simulink model "Testerr"  (R2024a)
settings: Solver=FixedStepAuto  StartTime=0.0  StopTime=inf  RelTol=1e-3  EnableMultiTasking=on
undefined symbols (not defined in the file): DiscIntNeverNeededParam
libraries: stm32f4xxblockslib x15, mcbpositiondecoderlib x4, stm32blockslib x3, simulink x1, mcbcontrolslib x1
settings Model: SimulationMode=external  Creator=wsl  LastModifiedBy=wsl
settings SolverCC: AllowMultiTaskInputOutput=on  AutoInsertRateTranBlk=on  InsertRTBMode=Never (minimum delay)
settings OptimizationCC: EnhancedBackFolding=on  PassReuseOutputArgsAs=Individual arguments  ZeroExternalMemoryAtStartup=off  ZeroInternalMemoryAtStartup=off  MaxStackSize=64  OptimizeBlockOrder=speed  DifferentSizesBufferReuse=on  OptimizationCustomize=off  EfficientTunableParamExpr=on
settings DebuggingCC: MultiTaskDSMMsg=none  TasksWithSamePriorityMsg=none  ParameterPrecisionLossMsg=none  ParameterTunabilityLossMsg=error
settings HardwareCC: ProdBitPerPointer=32  ProdBitPerSizeT=32  ProdBitPerPtrDiffT=32  ProdLargestAtomicInteger=Long  ProdLargestAtomicFloat=Double  ProdWordSize=32  ProdLongLongMode=on  ProdHWDeviceType=ARM Compatible->ARM Cortex-M
settings SFSimCC: MATLABDynamicMemAlloc=off
settings RTWCC: Description=Embedded Coder  SystemTargetFile=ert.tlc  HardwareBoard=STM32F4xx Based  TemplateMakefile=ert_default_tmf  Toolchain=GNU Tools for ARM Embedded Processors
settings CodeAppCC: ForceParamTrailComments=on  IgnoreCustomStorageClasses=off  OperatorAnnotations=on  SimulinkDataObjDesc=on  SFDataObjDesc=on  InsertBlockDesc=on
settings ERTTargetCC: TargetLangStandard=C99 (ISO)  CodeReplacementLibrary=ARM Cortex-M  ExtModeTransport=3  ExtModeStaticAlloc=on  ExtModeStaticAllocSize=2048  ExtModeMexFile=ext_xcp  ExtModeIntrfLevel=Level2 - Open

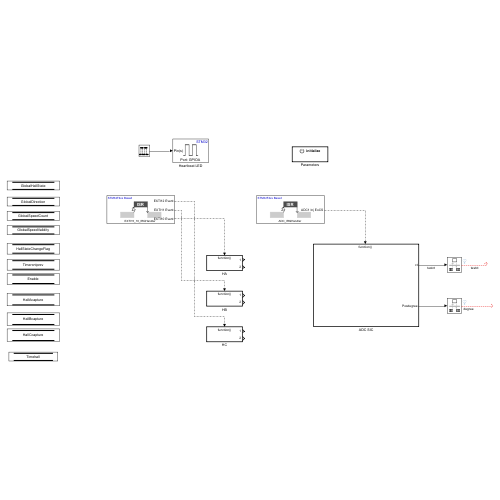
[thumbnail: Simulink's stored preview of the top-level diagram]
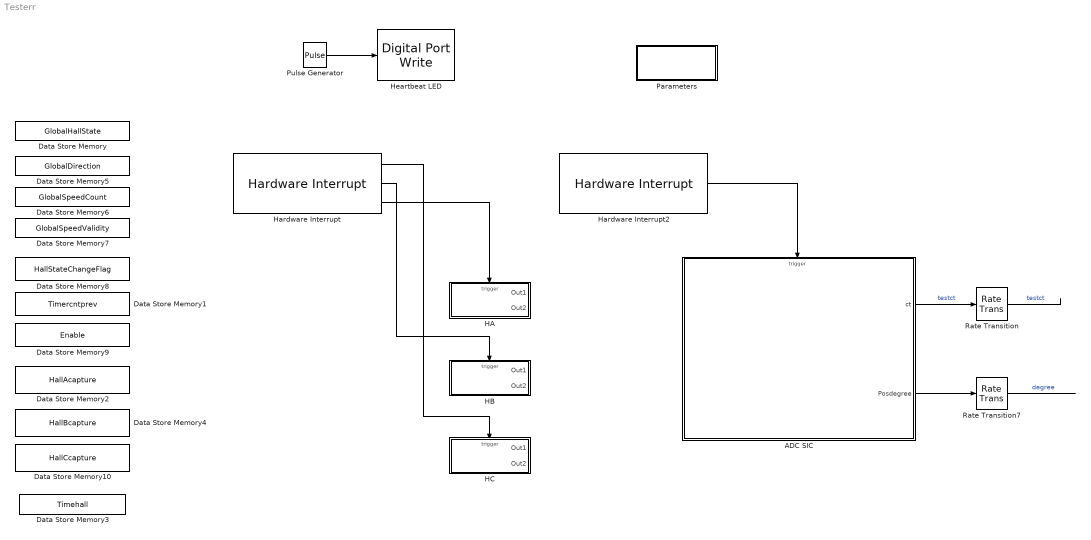
== system Testerr ==
  ADC SIC : Subsystem  TreatAsAtomicUnit=on
  Data Store Memory : DataStoreMemory  DataStoreName=GlobalHallState  WriteAfterWriteMsg=warning  ShowAdditionalParam=off
  Data Store Memory1 : DataStoreMemory  DataStoreName=Timercntprev  WriteAfterWriteMsg=warning  ShowAdditionalParam=off
  Data Store Memory10 : DataStoreMemory  DataStoreName=HallCcapture  WriteAfterWriteMsg=warning  ShowAdditionalParam=off
  Data Store Memory2 : DataStoreMemory  DataStoreName=HallAcapture  WriteAfterWriteMsg=warning  ShowAdditionalParam=off
  Data Store Memory3 : DataStoreMemory  DataStoreName=Timehall  WriteAfterWriteMsg=warning  ShowAdditionalParam=off
  Data Store Memory4 : DataStoreMemory  DataStoreName=HallBcapture  WriteAfterWriteMsg=warning  ShowAdditionalParam=off
  Data Store Memory5 : DataStoreMemory  DataStoreName=GlobalDirection  WriteAfterWriteMsg=warning  ShowAdditionalParam=off
  Data Store Memory6 : DataStoreMemory  DataStoreName=GlobalSpeedCount  WriteAfterWriteMsg=warning  ShowAdditionalParam=off
  Data Store Memory7 : DataStoreMemory  DataStoreName=GlobalSpeedValidity  WriteAfterWriteMsg=warning  ShowAdditionalParam=off
  Data Store Memory8 : DataStoreMemory  DataStoreName=HallStateChangeFlag  WriteAfterWriteMsg=warning  ShowAdditionalParam=off
  Data Store Memory9 : DataStoreMemory  DataStoreName=Enable  WriteAfterWriteMsg=warning  ShowAdditionalParam=off
  HA : Subsystem  TreatAsAtomicUnit=on
  HB : Subsystem  TreatAsAtomicUnit=on
  HC : Subsystem  TreatAsAtomicUnit=on
  Hardware Interrupt : stm32f4xxblockslib/Hardware Interrupt  ISRGroup=External interrupts (EXTI)  ISRName=EXTI15_10_IRQHandler  ISRNumber=55  EventsList={ 'off', 'EXTI15 Event', '1'; 'off', 'EXTI14 Event', '2'; 'off', 'EXTI13 Event', '3'; 'on', 'EXTI12 Event', '4'; 'on', 'EXTI11 Event', '5'; 'on', 'EXTI10 Event', '6'; 'off', 'Custom event', '7' }  SelectedEvents={'EXTI12 Event','EXTI11 Event','EXTI10 Event'}  TaskPriority=30  DisablePreemption=on  ClearInterruptFlagsAtEndOfEvent=off  InterruptDefinitionFile=$(TARGET_ROOT)/registry/interrupts/STM32F4xxBased_interrupts.xml  HardwareBoard=STM32F4xx Based  EnableSimPort=off
  Hardware Interrupt2 : stm32f4xxblockslib/Hardware Interrupt  ISRGroup=Analog to digital converter (ADC)  ISRName=ADC_IRQHandler  ISRNumber=33  EventsList={ 'off', 'ADC1 OVR', '1'; 'off', 'ADC1 Reg EoCS', '2'; 'on', 'ADC1 Inj EoCS', '3'; 'off', 'ADC1 Watchdog', '4'; 'off', 'ADC2 OVR', '5'; 'off', 'ADC2 Reg EoCS', '6'; 'off', 'ADC2 Inj EoCS', '7'; 'off', 'ADC2 Watchdog', '8'; 'off', 'ADC3 OVR', '9'; 'off', 'ADC3 Reg EoCS', '10'; 'off', 'ADC3 Inj EoCS', '11'; 'off', 'ADC3 Watchdog', '12'; 'off', 'Custom event', '13' }  SelectedEvents={'ADC1 Inj EoCS'}  TaskPriority=30  DisablePreemption=on  ClearInterruptFlagsAtEndOfEvent=off  InterruptDefinitionFile=$(TARGET_ROOT)/registry/interrupts/STM32F4xxBased_interrupts.xml  HardwareBoard=STM32F4xx Based  EnableSimPort=off
  Heartbeat LED : stm32f4xxblockslib/Digital Port Write  PortName=GPIOA  PinNumber=[5]  ReadOperation=off  IOAsArray=on  EnableSimPort=off
  Parameters : Subsystem  TreatAsAtomicUnit=on
  Pulse Generator : DiscretePulseGenerator  Period=10  PulseWidth=5  SampleTime=0.1
  Rate Transition : RateTransition  Deterministic=off  OutPortSampleTime=1e-3
  Rate Transition7 : RateTransition  Deterministic=off  OutPortSampleTime=1e-3
  wires:
  Pulse Generator/1 -> Heartbeat LED/1
  Hardware Interrupt/2 -> HB/Trigger
  Hardware Interrupt/3 -> HA/Trigger
  Hardware Interrupt/1 -> HC/Trigger
  Hardware Interrupt2/1 -> ADC SIC/Trigger
  ADC SIC/1(ct) -> Rate Transition/1  "testct"
  Rate Transition/1 -> ?  "testct"
  Rate Transition7/1 -> ?  "degree"
  ADC SIC/2(Posdegree) -> Rate Transition7/1

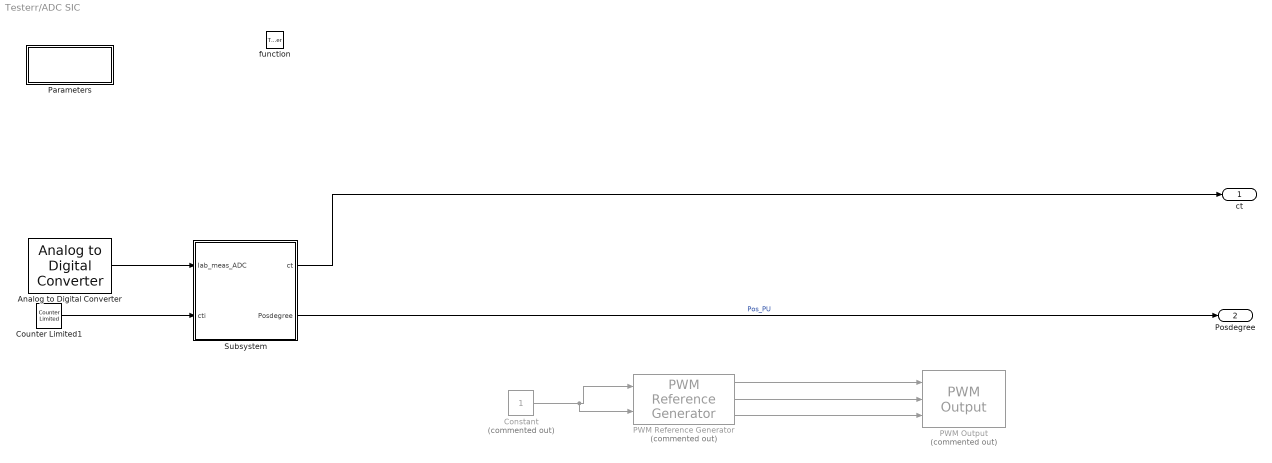
== system Testerr/ADC SIC ==
  function : TriggerPort  TriggerType=function-call  VariantControl=(inherit)
  Analog to Digital Converter : stm32f4xxblockslib/Analog to Digital Converter  ADCModule=ADC1  ConversionGroup=Injected  TriggerMode=Read results only  NumberOfConversions=3  EnableBufferConv=off  BufferLength=1  OutputStatus=off  SampleTime=-1  EnableSimPort=off
  Constant : Constant  Commented=on
  Counter Limited1 : simulink/Sources/Counter Limited  uplimit=20000  tsamp=-1
  PWM Output : stm32f4xxblockslib/PWM Output  Commented=on  TimerModule=TIM1  DutycycleUnits=Percentage  EnableChannel1=on  EnableChannel2=on  EnableChannel3=on  EnableChannel4=off  EnableCounterInput=off  EnableMainOutputInput=off  EnableFrequencyInput=off  SetRCAfterCE=on  OutputDirection=off  OutputMainOutputEnableStatus=off  SampleTime=0.1  EnableSimPort=off  EnableUpdateEvent=off  EnableCaptureCompare1Event=off  EnableCaptureCompare2Event=off  EnableCaptureCompare3Event=off  EnableCaptureCompare4Event=off  EnableTriggerEvent=off  EnableBreakEvent=off  ProcessorFamily=STM32F4  hoistedMaskSrc=ECSoC/ECSimCodegen/PWM Output
  PWM Reference Generator : mcbcontrolslib/PWM Reference Generator  Commented=on  inSignal=Valphabeta  modType=SVM: space vector modulation
      settings: LibrarySourceBlock=mcblib/Controls/Math Transforms/PWM Reference Generator
  Parameters : Subsystem  TreatAsAtomicUnit=on
  Subsystem : Subsystem
  ct : Outport
  Posdegree : Outport  Port=2
  wires:
  Analog to Digital Converter/1 -> Subsystem/1(Iab_meas_ADC)
  Counter Limited1/1 -> Subsystem/2(cti)
  Subsystem/1(ct) -> ct/1
  Subsystem/2(Posdegree) -> Posdegree/1  "Pos_PU"
  PWM Reference Generator/2 -> PWM Output/2
  PWM Reference Generator/1 -> PWM Output/1
  PWM Reference Generator/3 -> PWM Output/3
  Constant/1 -> PWM Reference Generator/2, PWM Reference Generator/1

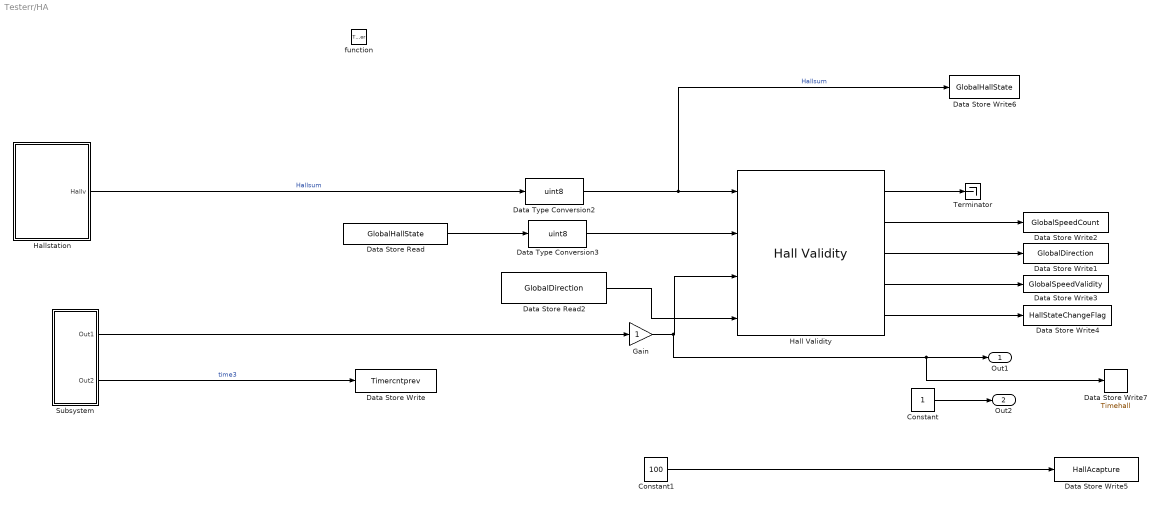
== system Testerr/HA ==
  function : TriggerPort  TriggerType=function-call  VariantControl=(inherit)
  Constant : Constant
  Constant1 : Constant  Value=100
  Data Store Read : DataStoreRead  DataStoreName=GlobalHallState  IndexOptions=Index vector (dialog)  Indices=1  OutputSizes=1
  Data Store Read2 : DataStoreRead  DataStoreName=GlobalDirection  IndexOptions=Index vector (dialog)  Indices=1  OutputSizes=1
  Data Store Write : DataStoreWrite  DataStoreName=Timercntprev  IndexOptions=Index vector (dialog)  Indices=1  OutputSizes=1
  Data Store Write1 : DataStoreWrite  DataStoreName=GlobalDirection  IndexOptions=Index vector (dialog)  Indices=1  OutputSizes=1
  Data Store Write2 : DataStoreWrite  DataStoreName=GlobalSpeedCount  IndexOptions=Index vector (dialog)  Indices=1  OutputSizes=1
  Data Store Write3 : DataStoreWrite  DataStoreName=GlobalSpeedValidity  IndexOptions=Index vector (dialog)  Indices=1  OutputSizes=1
  Data Store Write4 : DataStoreWrite  DataStoreName=HallStateChangeFlag  IndexOptions=Index vector (dialog)  Indices=1  OutputSizes=1
  Data Store Write5 : DataStoreWrite  DataStoreName=HallAcapture  IndexOptions=Index vector (dialog)  Indices=1  OutputSizes=1
  Data Store Write6 : DataStoreWrite  DataStoreName=GlobalHallState  IndexOptions=Index vector (dialog)  Indices=1  OutputSizes=1
  Data Store Write7 : DataStoreWrite  DataStoreName=Timehall  IndexOptions=Index vector (dialog)  Indices=1  OutputSizes=1
  Data Type Conversion2 : DataTypeConversion  OutDataTypeStr=uint8  SaturateOnIntegerOverflow=off  RndMeth=Floor
  Data Type Conversion3 : DataTypeConversion  OutDataTypeStr=uint8  SaturateOnIntegerOverflow=off  RndMeth=Floor
  Gain : Gain
  Hall Validity : mcbpositiondecoderlib/Hall Validity  hallSequence=ABC  sequence=[5,4,6,2,3,1]  CounterSize=32 bits
  Hallstation : Subsystem
  Subsystem : Subsystem
  Terminator : Terminator
  Out1 : Outport
  Out2 : Outport  Port=2
  wires:
  Hall Validity/2 -> Data Store Write2/1
  Hall Validity/3 -> Data Store Write1/1
  Data Store Read2/1 -> Hall Validity/4
  Hall Validity/1 -> Terminator/1
  Hall Validity/4 -> Data Store Write3/1
  Hall Validity/5 -> Data Store Write4/1
  Constant/1 -> Out2/1
  Data Store Read/1 -> Data Type Conversion3/1
  Hallstation/1(Hallv) -> Data Type Conversion2/1  "Hallsum"
  Data Type Conversion3/1 -> Hall Validity/2
  Subsystem/1(Out1) -> Gain/1
  Data Type Conversion2/1 -> Data Store Write6/1, Hall Validity/1  "Hallsum"
  Gain/1 -> Data Store Write7/1, Out1/1, Hall Validity/3
  Constant1/1 -> Data Store Write5/1
  Subsystem/2(Out2) -> Data Store Write/1  "time3"

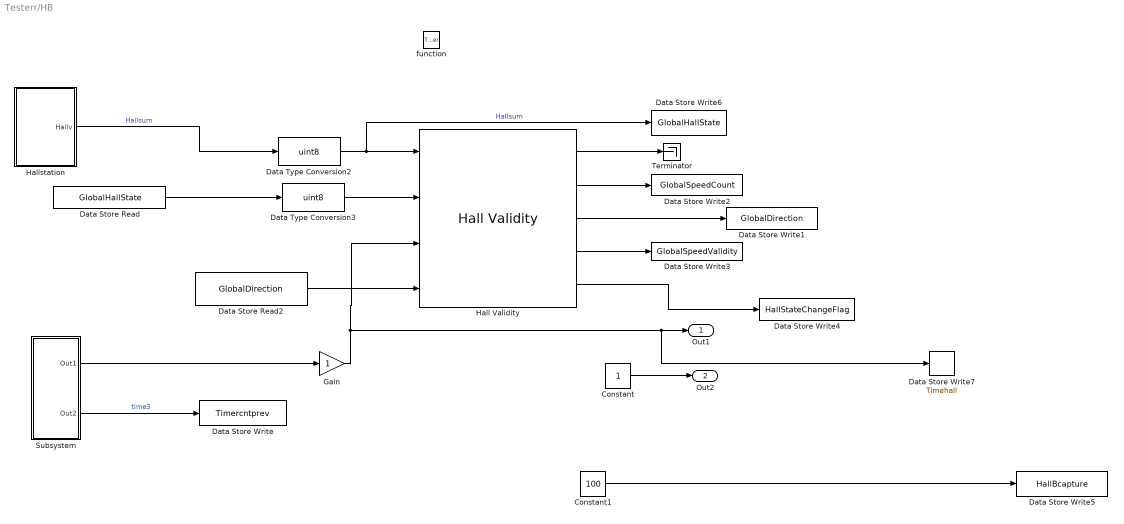
== system Testerr/HB ==
  function : TriggerPort  TriggerType=function-call  VariantControl=(inherit)
  Constant : Constant
  Constant1 : Constant  Value=100
  Data Store Read : DataStoreRead  DataStoreName=GlobalHallState  IndexOptions=Index vector (dialog)  Indices=1  OutputSizes=1
  Data Store Read2 : DataStoreRead  DataStoreName=GlobalDirection  IndexOptions=Index vector (dialog)  Indices=1  OutputSizes=1
  Data Store Write : DataStoreWrite  DataStoreName=Timercntprev  IndexOptions=Index vector (dialog)  Indices=1  OutputSizes=1
  Data Store Write1 : DataStoreWrite  DataStoreName=GlobalDirection  IndexOptions=Index vector (dialog)  Indices=1  OutputSizes=1
  Data Store Write2 : DataStoreWrite  DataStoreName=GlobalSpeedCount  IndexOptions=Index vector (dialog)  Indices=1  OutputSizes=1
  Data Store Write3 : DataStoreWrite  DataStoreName=GlobalSpeedValidity  IndexOptions=Index vector (dialog)  Indices=1  OutputSizes=1
  Data Store Write4 : DataStoreWrite  DataStoreName=HallStateChangeFlag  IndexOptions=Index vector (dialog)  Indices=1  OutputSizes=1
  Data Store Write5 : DataStoreWrite  DataStoreName=HallBcapture  IndexOptions=Index vector (dialog)  Indices=1  OutputSizes=1
  Data Store Write6 : DataStoreWrite  DataStoreName=GlobalHallState  IndexOptions=Index vector (dialog)  Indices=1  OutputSizes=1
  Data Store Write7 : DataStoreWrite  DataStoreName=Timehall  IndexOptions=Index vector (dialog)  Indices=1  OutputSizes=1
  Data Type Conversion2 : DataTypeConversion  OutDataTypeStr=uint8  SaturateOnIntegerOverflow=off  RndMeth=Floor
  Data Type Conversion3 : DataTypeConversion  OutDataTypeStr=uint8  SaturateOnIntegerOverflow=off  RndMeth=Floor
  Gain : Gain
  Hall Validity : mcbpositiondecoderlib/Hall Validity  hallSequence=ABC  sequence=[5,4,6,2,3,1]  CounterSize=32 bits
  Hallstation : Subsystem
  Subsystem : Subsystem
  Terminator : Terminator
  Out1 : Outport
  Out2 : Outport  Port=2
  wires:
  Hall Validity/2 -> Data Store Write2/1
  Hall Validity/3 -> Data Store Write1/1
  Data Store Read2/1 -> Hall Validity/4
  Hall Validity/1 -> Terminator/1
  Hall Validity/4 -> Data Store Write3/1
  Hall Validity/5 -> Data Store Write4/1
  Constant/1 -> Out2/1
  Hallstation/1(Hallv) -> Data Type Conversion2/1  "Hallsum"
  Data Type Conversion3/1 -> Hall Validity/2
  Subsystem/1(Out1) -> Gain/1
  Data Type Conversion2/1 -> Data Store Write6/1, Hall Validity/1  "Hallsum"
  Data Store Read/1 -> Data Type Conversion3/1
  Gain/1 -> Hall Validity/3, Data Store Write7/1, Out1/1
  Constant1/1 -> Data Store Write5/1
  Subsystem/2(Out2) -> Data Store Write/1  "time3"

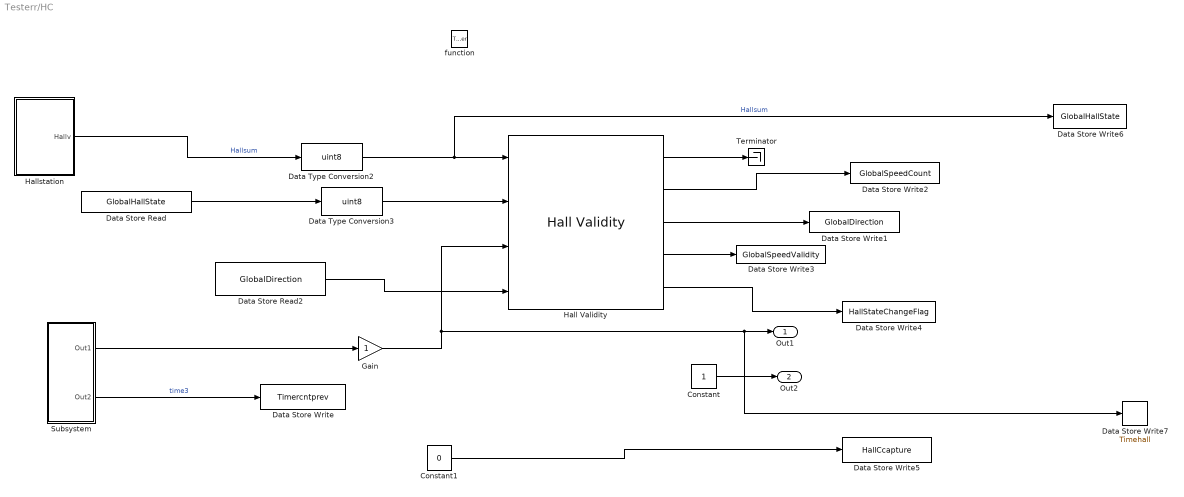
== system Testerr/HC ==
  function : TriggerPort  TriggerType=function-call  VariantControl=(inherit)
  Constant : Constant
  Constant1 : Constant  Value=0
  Data Store Read : DataStoreRead  DataStoreName=GlobalHallState  IndexOptions=Index vector (dialog)  Indices=1  OutputSizes=1
  Data Store Read2 : DataStoreRead  DataStoreName=GlobalDirection  IndexOptions=Index vector (dialog)  Indices=1  OutputSizes=1
  Data Store Write : DataStoreWrite  DataStoreName=Timercntprev  IndexOptions=Index vector (dialog)  Indices=1  OutputSizes=1
  Data Store Write1 : DataStoreWrite  DataStoreName=GlobalDirection  IndexOptions=Index vector (dialog)  Indices=1  OutputSizes=1
  Data Store Write2 : DataStoreWrite  DataStoreName=GlobalSpeedCount  IndexOptions=Index vector (dialog)  Indices=1  OutputSizes=1
  Data Store Write3 : DataStoreWrite  DataStoreName=GlobalSpeedValidity  IndexOptions=Index vector (dialog)  Indices=1  OutputSizes=1
  Data Store Write4 : DataStoreWrite  DataStoreName=HallStateChangeFlag  IndexOptions=Index vector (dialog)  Indices=1  OutputSizes=1
  Data Store Write5 : DataStoreWrite  DataStoreName=HallCcapture  IndexOptions=Index vector (dialog)  Indices=1  OutputSizes=1
  Data Store Write6 : DataStoreWrite  DataStoreName=GlobalHallState  IndexOptions=Index vector (dialog)  Indices=1  OutputSizes=1
  Data Store Write7 : DataStoreWrite  DataStoreName=Timehall  IndexOptions=Index vector (dialog)  Indices=1  OutputSizes=1
  Data Type Conversion2 : DataTypeConversion  OutDataTypeStr=uint8  SaturateOnIntegerOverflow=off  RndMeth=Floor
  Data Type Conversion3 : DataTypeConversion  OutDataTypeStr=uint8  SaturateOnIntegerOverflow=off  RndMeth=Floor
  Gain : Gain
  Hall Validity : mcbpositiondecoderlib/Hall Validity  hallSequence=ABC  sequence=[5,4,6,2,3,1]  CounterSize=32 bits
  Hallstation : Subsystem
  Subsystem : Subsystem
  Terminator : Terminator
  Out1 : Outport
  Out2 : Outport  Port=2
  wires:
  Hall Validity/2 -> Data Store Write2/1
  Hall Validity/3 -> Data Store Write1/1
  Data Store Read2/1 -> Hall Validity/4
  Hall Validity/1 -> Terminator/1
  Hall Validity/4 -> Data Store Write3/1
  Hall Validity/5 -> Data Store Write4/1
  Constant/1 -> Out2/1
  Hallstation/1(Hallv) -> Data Type Conversion2/1  "Hallsum"
  Data Store Read/1 -> Data Type Conversion3/1
  Subsystem/1(Out1) -> Gain/1
  Data Type Conversion3/1 -> Hall Validity/2
  Data Type Conversion2/1 -> Data Store Write6/1, Hall Validity/1  "Hallsum"
  Gain/1 -> Hall Validity/3, Data Store Write7/1, Out1/1
  Constant1/1 -> Data Store Write5/1
  Subsystem/2(Out2) -> Data Store Write/1  "time3"

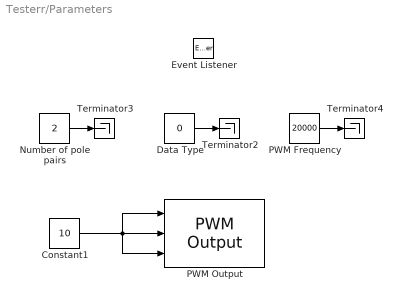
== system Testerr/Parameters ==
  Constant1 : Constant  Value=10  VectorParams1D=off
  Data Type : Constant  Value=0
  Event Listener : EventListener  DisableCoverage=on  EventName=reset
  Number of pole pairs : Constant  Value=2
  PWM Frequency : Constant  Value=20000
  PWM Output : stm32f4xxblockslib/PWM Output  TimerModule=TIM1  DutycycleUnits=Percentage  EnableChannel1=on  EnableChannel2=on  EnableChannel3=on  EnableChannel4=off  EnableCounterInput=off  EnableMainOutputInput=off  EnableFrequencyInput=off  SetRCAfterCE=on  OutputDirection=off  OutputMainOutputEnableStatus=off  SampleTime=0.1  EnableSimPort=off  EnableUpdateEvent=off  EnableCaptureCompare1Event=off  EnableCaptureCompare2Event=off  EnableCaptureCompare3Event=off  EnableCaptureCompare4Event=off  EnableTriggerEvent=off  EnableBreakEvent=off  ProcessorFamily=STM32F4  hoistedMaskSrc=ECSoC/ECSimCodegen/PWM Output
  Terminator2 : Terminator
  Terminator3 : Terminator
  Terminator4 : Terminator
  wires:
  PWM Frequency/1 -> Terminator4/1
  Number of pole pairs/1 -> Terminator3/1
  Data Type/1 -> Terminator2/1
  Constant1/1 -> PWM Output/3, PWM Output/2, PWM Output/1

== system Testerr/ADC SIC/Parameters ==
  Data Type : Constant  Value=0
  Event Listener : EventListener  DisableCoverage=on  EventName=reset
  Number of pole pairs : Constant  Value=4
  PWM Frequency : Constant  Value=20000
  Terminator2 : Terminator
  Terminator3 : Terminator
  Terminator4 : Terminator
  wires:
  PWM Frequency/1 -> Terminator4/1
  Number of pole pairs/1 -> Terminator3/1
  Data Type/1 -> Terminator2/1

== system Testerr/ADC SIC/Subsystem ==
  Iab_meas_ADC : Inport  OutDataTypeStr=uint16
  cti : Inport  Port=2
  Subsystem1 : Subsystem
  Terminator : Terminator
  ct : Outport
  Posdegree : Outport  Port=2
  wires:
  Iab_meas_ADC/1 -> Terminator/1
  Subsystem1/2(Posdegree) -> Posdegree/1
  Subsystem1/1(ct) -> ct/1
  cti/1 -> Subsystem1/1(cti)

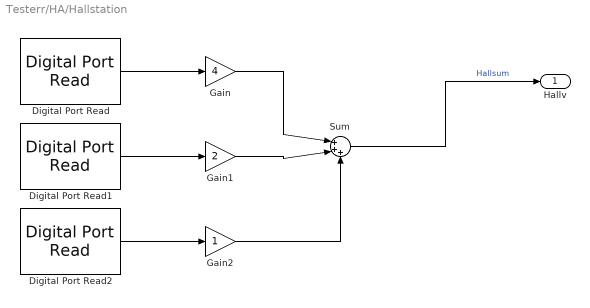
== system Testerr/HA/Hallstation ==
  Digital Port Read : stm32f4xxblockslib/Digital Port Read  PortName=GPIOC  PinNumber=[10]  ReadOperation=on  IOAsArray=on  SampleTime=-1  EnableSimPort=off
  Digital Port Read1 : stm32f4xxblockslib/Digital Port Read  PortName=GPIOC  PinNumber=[11]  ReadOperation=on  IOAsArray=on  SampleTime=-1  EnableSimPort=off
  Digital Port Read2 : stm32f4xxblockslib/Digital Port Read  PortName=GPIOC  PinNumber=[12]  ReadOperation=on  IOAsArray=on  SampleTime=-1  EnableSimPort=off
  Gain : Gain  Gain=4  OutDataTypeStr=uint8
  Gain1 : Gain  Gain=2  OutDataTypeStr=uint8
  Gain2 : Gain  OutDataTypeStr=uint8
  Sum : Sum  Inputs=|+++
  Hallv : Outport
  wires:
  Digital Port Read1/1 -> Gain1/1
  Digital Port Read2/1 -> Gain2/1
  Digital Port Read/1 -> Gain/1
  Gain2/1 -> Sum/3
  Gain1/1 -> Sum/2
  Gain/1 -> Sum/1
  Sum/1 -> Hallv/1  "Hallsum"

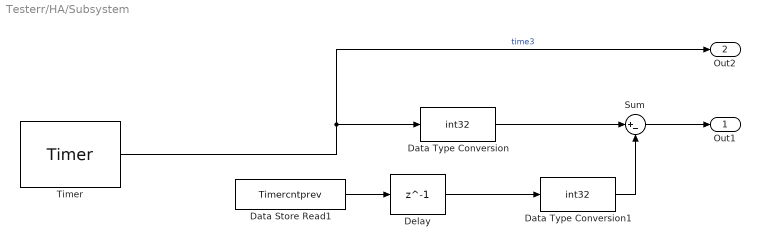
== system Testerr/HA/Subsystem ==
  Data Store Read1 : DataStoreRead  DataStoreName=Timercntprev  IndexOptions=Index vector (dialog)  Indices=1  OutputSizes=1
  Data Type Conversion : DataTypeConversion  OutDataTypeStr=int32  SaturateOnIntegerOverflow=off  RndMeth=Floor
  Data Type Conversion1 : DataTypeConversion  OutDataTypeStr=int32  SaturateOnIntegerOverflow=off  RndMeth=Floor
  Delay : Delay  DelayLength=1  InitialCondition=0  UseCircularBuffer=on
  Sum : Sum  Inputs=|+-
  Timer : stm32blockslib/Timer  TimerModule=TIM2  EnableFrequencyInput=off  EnableCounterInput=off  EnableMainOutputInput=off  SetRCAfterCE=off  OutputDirection=off  OutputMainOutputEnableStatus=off  SampleTime=-1  EnableUpdateEvent=off  EnableCaptureCompare1Event=off  EnableCaptureCompare2Event=off  EnableCaptureCompare3Event=off  EnableCaptureCompare4Event=off  EnableTriggerEvent=off  EnableBreakEvent=off  EnableBreakEvent2=off  EnableCOMGenerationEvent=off  ProcessorFamily=STM32F7
      settings: LibrarySourceBlock=stm32f4xxblockslib/Timer
  Out1 : Outport
  Out2 : Outport  Port=2
  wires:
  Sum/1 -> Out1/1
  Data Type Conversion/1 -> Sum/1
  Timer/1 -> Data Type Conversion/1, Out2/1  "time3"
  Data Store Read1/1 -> Delay/1
  Delay/1 -> Data Type Conversion1/1
  Data Type Conversion1/1 -> Sum/2

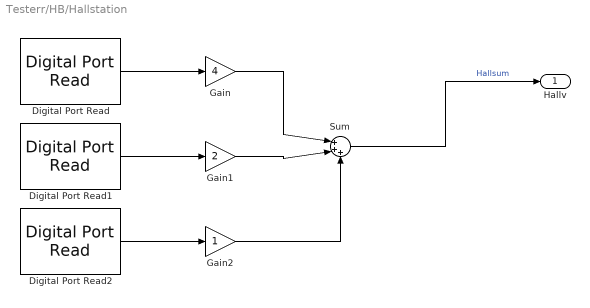
== system Testerr/HB/Hallstation ==
  Digital Port Read : stm32f4xxblockslib/Digital Port Read  PortName=GPIOC  PinNumber=[10]  ReadOperation=on  IOAsArray=on  SampleTime=-1  EnableSimPort=off
  Digital Port Read1 : stm32f4xxblockslib/Digital Port Read  PortName=GPIOC  PinNumber=[11]  ReadOperation=on  IOAsArray=on  SampleTime=-1  EnableSimPort=off
  Digital Port Read2 : stm32f4xxblockslib/Digital Port Read  PortName=GPIOC  PinNumber=[12]  ReadOperation=on  IOAsArray=on  SampleTime=-1  EnableSimPort=off
  Gain : Gain  Gain=4  OutDataTypeStr=uint8
  Gain1 : Gain  Gain=2  OutDataTypeStr=uint8
  Gain2 : Gain  OutDataTypeStr=uint8
  Sum : Sum  Inputs=|+++
  Hallv : Outport
  wires:
  Digital Port Read1/1 -> Gain1/1
  Digital Port Read2/1 -> Gain2/1
  Digital Port Read/1 -> Gain/1
  Gain2/1 -> Sum/3
  Gain1/1 -> Sum/2
  Gain/1 -> Sum/1
  Sum/1 -> Hallv/1  "Hallsum"

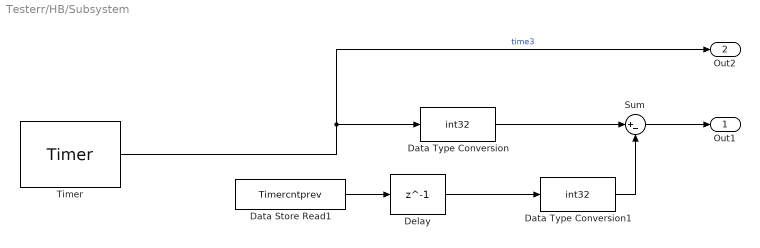
== system Testerr/HB/Subsystem ==
  Data Store Read1 : DataStoreRead  DataStoreName=Timercntprev  IndexOptions=Index vector (dialog)  Indices=1  OutputSizes=1
  Data Type Conversion : DataTypeConversion  OutDataTypeStr=int32  SaturateOnIntegerOverflow=off  RndMeth=Floor
  Data Type Conversion1 : DataTypeConversion  OutDataTypeStr=int32  SaturateOnIntegerOverflow=off  RndMeth=Floor
  Delay : Delay  DelayLength=1  InitialCondition=0  UseCircularBuffer=on
  Sum : Sum  Inputs=|+-
  Timer : stm32blockslib/Timer  TimerModule=TIM2  EnableFrequencyInput=off  EnableCounterInput=off  EnableMainOutputInput=off  SetRCAfterCE=off  OutputDirection=off  OutputMainOutputEnableStatus=off  SampleTime=-1  EnableUpdateEvent=off  EnableCaptureCompare1Event=off  EnableCaptureCompare2Event=off  EnableCaptureCompare3Event=off  EnableCaptureCompare4Event=off  EnableTriggerEvent=off  EnableBreakEvent=off  EnableBreakEvent2=off  EnableCOMGenerationEvent=off  ProcessorFamily=STM32F7
      settings: LibrarySourceBlock=stm32f4xxblockslib/Timer
  Out1 : Outport
  Out2 : Outport  Port=2
  wires:
  Sum/1 -> Out1/1
  Data Type Conversion/1 -> Sum/1
  Timer/1 -> Data Type Conversion/1, Out2/1  "time3"
  Data Store Read1/1 -> Delay/1
  Delay/1 -> Data Type Conversion1/1
  Data Type Conversion1/1 -> Sum/2

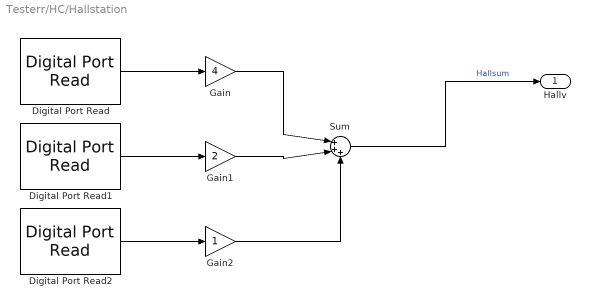
== system Testerr/HC/Hallstation ==
  Digital Port Read : stm32f4xxblockslib/Digital Port Read  PortName=GPIOC  PinNumber=[10]  ReadOperation=on  IOAsArray=on  SampleTime=-1  EnableSimPort=off
  Digital Port Read1 : stm32f4xxblockslib/Digital Port Read  PortName=GPIOC  PinNumber=[11]  ReadOperation=on  IOAsArray=on  SampleTime=-1  EnableSimPort=off
  Digital Port Read2 : stm32f4xxblockslib/Digital Port Read  PortName=GPIOC  PinNumber=[12]  ReadOperation=on  IOAsArray=on  SampleTime=-1  EnableSimPort=off
  Gain : Gain  Gain=4  OutDataTypeStr=uint8
  Gain1 : Gain  Gain=2  OutDataTypeStr=uint8
  Gain2 : Gain  OutDataTypeStr=uint8
  Sum : Sum  Inputs=|+++
  Hallv : Outport
  wires:
  Digital Port Read1/1 -> Gain1/1
  Digital Port Read2/1 -> Gain2/1
  Digital Port Read/1 -> Gain/1
  Gain2/1 -> Sum/3
  Gain1/1 -> Sum/2
  Gain/1 -> Sum/1
  Sum/1 -> Hallv/1  "Hallsum"

== system Testerr/HC/Subsystem ==
  Data Store Read1 : DataStoreRead  DataStoreName=Timercntprev  IndexOptions=Index vector (dialog)  Indices=1  OutputSizes=1
  Data Type Conversion : DataTypeConversion  OutDataTypeStr=int32  SaturateOnIntegerOverflow=off  RndMeth=Floor
  Data Type Conversion1 : DataTypeConversion  OutDataTypeStr=int32  SaturateOnIntegerOverflow=off  RndMeth=Floor
  Delay : Delay  DelayLength=1  InitialCondition=0  UseCircularBuffer=on
  Sum : Sum  Inputs=|+-
  Timer : stm32blockslib/Timer  TimerModule=TIM2  EnableFrequencyInput=off  EnableCounterInput=off  EnableMainOutputInput=off  SetRCAfterCE=off  OutputDirection=off  OutputMainOutputEnableStatus=off  SampleTime=-1  EnableUpdateEvent=off  EnableCaptureCompare1Event=off  EnableCaptureCompare2Event=off  EnableCaptureCompare3Event=off  EnableCaptureCompare4Event=off  EnableTriggerEvent=off  EnableBreakEvent=off  EnableBreakEvent2=off  EnableCOMGenerationEvent=off  ProcessorFamily=STM32F7
      settings: LibrarySourceBlock=stm32f4xxblockslib/Timer
  Out1 : Outport
  Out2 : Outport  Port=2
  wires:
  Sum/1 -> Out1/1
  Data Type Conversion/1 -> Sum/1
  Timer/1 -> Data Type Conversion/1, Out2/1  "time3"
  Data Store Read1/1 -> Delay/1
  Delay/1 -> Data Type Conversion1/1
  Data Type Conversion1/1 -> Sum/2

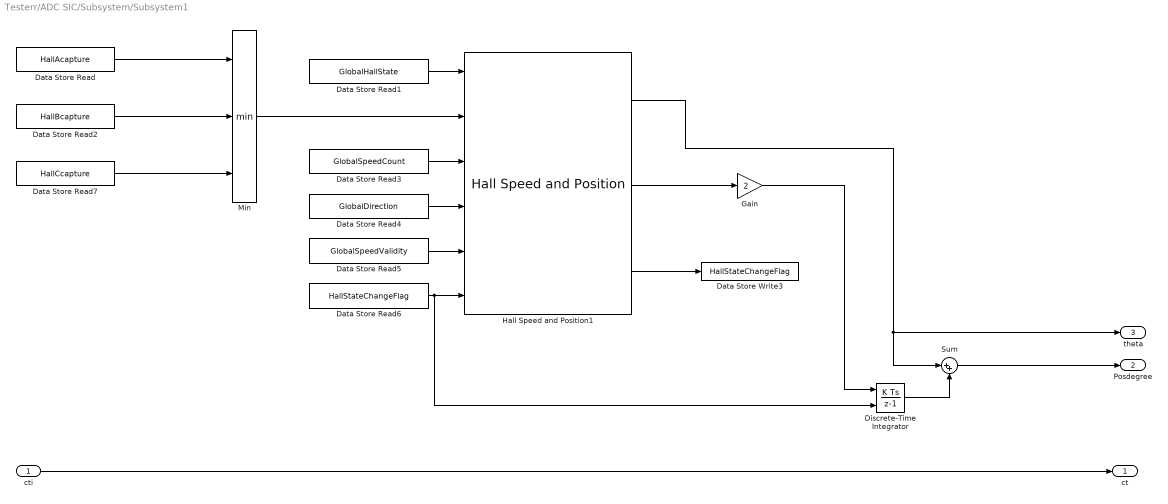
== system Testerr/ADC SIC/Subsystem/Subsystem1 ==
  cti : Inport
  Data Store Read : DataStoreRead  DataStoreName=HallAcapture  IndexOptions=Index vector (dialog)  Indices=1  OutputSizes=1
  Data Store Read1 : DataStoreRead  DataStoreName=GlobalHallState  IndexOptions=Index vector (dialog)  Indices=1  OutputSizes=1
  Data Store Read2 : DataStoreRead  DataStoreName=HallBcapture  IndexOptions=Index vector (dialog)  Indices=1  OutputSizes=1
  Data Store Read3 : DataStoreRead  DataStoreName=GlobalSpeedCount  IndexOptions=Index vector (dialog)  Indices=1  OutputSizes=1
  Data Store Read4 : DataStoreRead  DataStoreName=GlobalDirection  IndexOptions=Index vector (dialog)  Indices=1  OutputSizes=1
  Data Store Read5 : DataStoreRead  DataStoreName=GlobalSpeedValidity  IndexOptions=Index vector (dialog)  Indices=1  OutputSizes=1
  Data Store Read6 : DataStoreRead  Priority=1  DataStoreName=HallStateChangeFlag  IndexOptions=Index vector (dialog)  Indices=1  OutputSizes=1
  Data Store Read7 : DataStoreRead  DataStoreName=HallCcapture  IndexOptions=Index vector (dialog)  Indices=1  OutputSizes=1
  Data Store Write3 : DataStoreWrite  Priority=2  DataStoreName=HallStateChangeFlag  IndexOptions=Index vector (dialog)  Indices=1  OutputSizes=1
  Discrete-Time Integrator : DiscreteIntegrator  ExternalReset=rising  SampleTime=-1  LimitOutput=on  UpperSaturationLimit=60  LowerSaturationLimit=-60  ICPrevOutput=DiscIntNeverNeededParam  ICPrevScaledInput=DiscIntNeverNeededParam
  Gain : Gain  Gain=2
  Hall Speed and Position1 : mcbpositiondecoderlib/Hall Speed and Position  blkExecutionType=Speed and position  CounterSize=32 bits  ClkFreq=84e6  BlkSampleTime=5e-5  PolePairs=2  MinSpeed=20  HallInterruptConfig=Every 180 Degrees  SpeedUnit=Degrees/sec  PerUnitSpeed=6000  SpeedDataType=single  hallSequence=ABC  Sequence=[5,4,6,2,3,1]  EnableSecondOrder=1st Order  PositionUnit=Degrees  PositionDataType=dataType
  Min : MinMax  Inputs=3
  Sum : Sum  Inputs=|++
  ct : Outport
  Posdegree : Outport  Port=2  InitialOutput=0  VectorParamsAs1DForOutWhenUnconnected=off
  theta : Outport  Port=3  InitialOutput=0  VectorParamsAs1DForOutWhenUnconnected=off
  wires:
  Data Store Read/1 -> Min/1
  Data Store Read5/1 -> Hall Speed and Position1/5
  Data Store Read2/1 -> Min/2
  Data Store Read1/1 -> Hall Speed and Position1/1
  Data Store Read7/1 -> Min/3
  Data Store Read4/1 -> Hall Speed and Position1/4
  Min/1 -> Hall Speed and Position1/2
  Data Store Read3/1 -> Hall Speed and Position1/3
  Hall Speed and Position1/3 -> Data Store Write3/1
  cti/1 -> ct/1
  Data Store Read6/1 -> Discrete-Time Integrator/2, Hall Speed and Position1/6
  Hall Speed and Position1/2 -> Gain/1
  Discrete-Time Integrator/1 -> Sum/2
  Hall Speed and Position1/1 -> theta/1, Sum/1
  Sum/1 -> Posdegree/1
  Gain/1 -> Discrete-Time Integrator/1
